simulink model "ardupilotsailboatold"  (R2022b)
settings: Solver=VariableStepAuto  StartTime=0.0  StopTime=10.0  RelTol=1e-3
values from neighbouring files (symbols this model uses):
  Ixx = 1/120 * pi * rho * L * B * T * (4*T^2 + B^2)    (= 0.835683076278)    [parameterCalculations.m]
  m = 2    [parameterCalculations.m]
  m11 = m*k11    [parameterCalculations.m]
  m22 = m*k22    [parameterCalculations.m]
  Yv = Yv * (u^2)/(U^2)    (= -23.3298597446)    [parameterCalculations.m]
undefined symbols (not defined in the file or in its folder): Waypoints
libraries: cstblocks x2, simulink x1
settings Model: Creator=ruben  LastModifiedBy=ruben

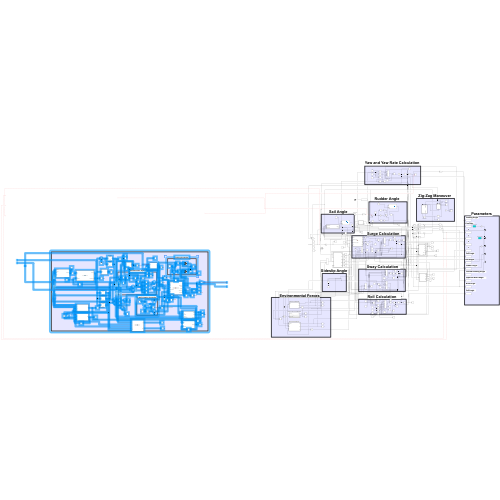
[thumbnail: Simulink's stored preview of the top-level diagram]
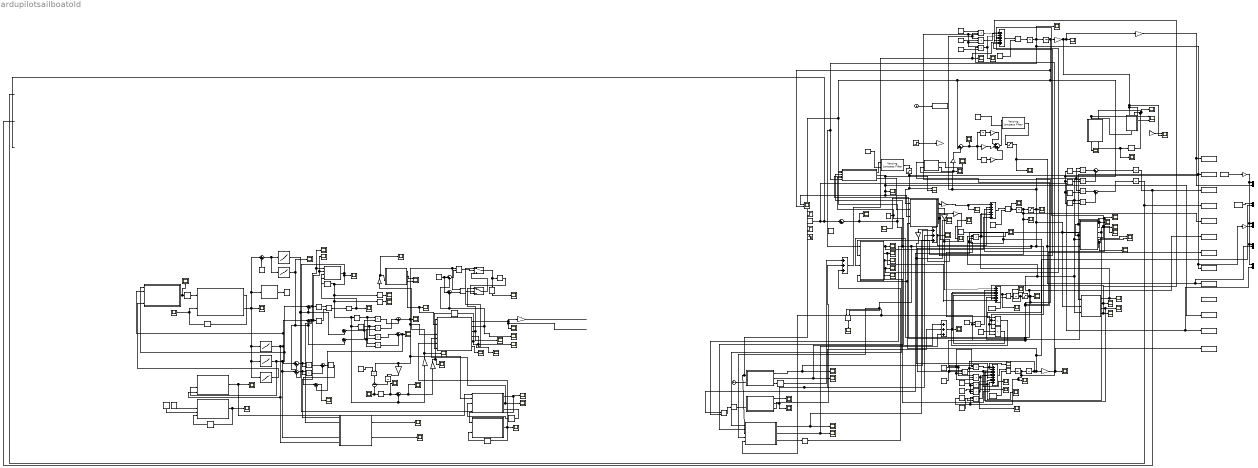
== system ardupilotsailboatold ==
  note: Yaw and Yaw Rate Calculation
  note: Surge Calculation
  note: Wave Forces and Moments
  note: Ocean Current Forces and Moments
  note: Sideslip Angle
  note: Parameters
  note: x
  note: Roll Calculation
  note: v
  note: Heading Angle
  note: u
  note: Roll Angle
  note: Sail Angle
  note: Sail Angle
  note: y
  note: Zig-Zag Maneuver
  note: Desired Heading Angle
  note: Environmental Forces
  note: Roll Angle
  note: Wind Forces and Moments
  note: Apparent Wind Angle
  note: Rudder Angle
  note: Wind Angle
  note: Sway Calculation
  note: Rudder Angle
  note: Yaw Rate
  note: Path Following Controller
  note: Tacking Controller
  note: Guidance Axis System
  Abs : Abs  SaturateOnIntegerOverflow=off
  Abs1 : Abs  SaturateOnIntegerOverflow=off
  Abs2 : Abs  SaturateOnIntegerOverflow=off
  Clock : Clock
  Clock1 : Clock
  Constant : Constant  Value=m11
  Constant1 : Constant  Value=m22
  Constant2 : Constant
  Constant27 : Constant  Value=0.1
  Constant3 : Constant  Value=-100
  Constant4 : Constant  Value=-8190/100
  Constant5 : Constant  Value=5.89/100
  Delay{1..2,4..7,9..12} (10 alike) : Delay  DelayLength=1
  Delay13 : Delay  DelayLength=1  SampleTime=2
  Delay14 : Delay  DelayLength=1  SampleTime=0.01
  Delay3 : Delay  DelayLength=1  SampleTime=2
  Derivative : Derivative
  Divide{,1..6} (7 alike) : Product  Inputs=*/
  Gain : Gain  Gain=0.9
  Gain1 : Gain  Gain=0.29
  Gain{3..4,10,17} (4 alike) : Gain  Gain=pi/180
  Gain12 : Gain  Gain=-1
  Gain{7..9,13} (4 alike) : Gain
  Gain{2,15..16,18} (4 alike) : Gain  Gain=180/pi
  Gain5 : Gain  Gain=0.01
  Gain6 : Gain  Gain=-180/pi
  Integrator{1..2,4..9} (8 alike) : Integrator
  Integrator17 : Integrator  LimitOutput=on  UpperSaturationLimit=10  LowerSaturationLimit=-10
  Integrator3 : Integrator  InitialCondition=1.3
  KS : Scope
  Kk : Scope
  Kr : Scope
  MATLAB Function : MATLAB Function  TreatAsAtomicUnit=on
  MATLAB Function1 : MATLAB Function  TreatAsAtomicUnit=on
  MATLAB Function10 : MATLAB Function  TreatAsAtomicUnit=on
  MATLAB Function11 : MATLAB Function  TreatAsAtomicUnit=on
  MATLAB Function12 : MATLAB Function  TreatAsAtomicUnit=on
  MATLAB Function13 : MATLAB Function  TreatAsAtomicUnit=on
  MATLAB Function14 : MATLAB Function  TreatAsAtomicUnit=on
  MATLAB Function15 : MATLAB Function  TreatAsAtomicUnit=on
  MATLAB Function16 : MATLAB Function  TreatAsAtomicUnit=on
  MATLAB Function18 : MATLAB Function  TreatAsAtomicUnit=on
  MATLAB Function19 : MATLAB Function  TreatAsAtomicUnit=on
  MATLAB Function2 : MATLAB Function  TreatAsAtomicUnit=on
  MATLAB Function20 : MATLAB Function  TreatAsAtomicUnit=on
  MATLAB Function21 : MATLAB Function  TreatAsAtomicUnit=on
  MATLAB Function3 : MATLAB Function  TreatAsAtomicUnit=on
  MATLAB Function4 : MATLAB Function  TreatAsAtomicUnit=on
  MATLAB Function5 : MATLAB Function  TreatAsAtomicUnit=on
  MATLAB Function6 : MATLAB Function  TreatAsAtomicUnit=on
  MATLAB Function7 : MATLAB Function  TreatAsAtomicUnit=on
  MATLAB Function8 : MATLAB Function  TreatAsAtomicUnit=on
  MATLAB Function9 : MATLAB Function  TreatAsAtomicUnit=on
  Memory : Memory
  Mux{2..6} (5 alike) : Mux  Inputs=2
  NS : Scope
  Nk : Scope
  Nr : Scope
  Product{,1..2,7..13,84..85,88} (13 alike) : Product
  Product{3..6,14..20} (11 alike) : Product  Inputs=3
  Radius of Acceptance R : Lookup_n-D  NumberOfTableDimensions=1  BreakpointsForDimension1=Waypoints.number  Table=Waypoints.R  InterpMethod=Cubic spline  ExtrapMethod=Cubic spline  InternalRulePriority=Speed  RndMeth=Simplest
  Relational Operator : RelationalOperator  Operator=<=  OutDataTypeStr=boolean  RndMeth=Simplest  InputSameDT=off
  Relational Operator1 : RelationalOperator  Operator=>  OutDataTypeStr=boolean  RndMeth=Simplest  InputSameDT=off
  Roll Axis of Rotation : Constant  Value=[ -1 0 0 ]
  Saturation : Saturate  UpperLimit=pi/6  LowerLimit=-pi/6  ZeroCross=off
  Saturation1 : Saturate  UpperLimit=1.3  LowerLimit=-1.3
  Saturation2 : Saturate  UpperLimit=pi/3  LowerLimit=-pi/3
  Saturation3 : Saturate  UpperLimit=0.1  LowerLimit=-0.1
  Scope{1,3..15,17..29,31..32,34} (30 alike) : Scope
  Scope16 : Scope  NumInputPorts=2
  Scope2 : Scope  NumInputPorts=2
  Scope30 : Scope  NumInputPorts=2
  Sine Wave : Sin  Amplitude=pi/4  Frequency=0.1  SampleTime=0
  Sqrt : Sqrt
  Step1 : Step  Time=0  After=pi-0.01  SampleTime=0
  Step2 : Step  Time=50  After=0  SampleTime=0
  Stop Simulation : Stop
  Subsystem : Subsystem
  Sum : Sum  Inputs=|+--
  Sum{1,13,15,17} (4 alike) : Sum  Inputs=|+++
  Sum{6,9..11} (4 alike) : Sum  Inputs=|+-
  Sum{7..8,14,18} (4 alike) : Sum  Inputs=|++
  Sum16 : Sum  Inputs=|--
  Sum19 : Sum  Inputs=|-+-+++++
  Sum3 : Sum  Inputs=|++++++
  Sum4 : Sum  Inputs=|+++-++++
  Sum5 : Sum  Inputs=|+-++++++++
  Tack Direction : Constant  Value=0
  Tack Left : Switch  Criteria=u2 > Threshold  SaturateOnIntegerOverflow=off  InputSameDT=off
  Tack Right : Switch  Criteria=u2 > Threshold  SaturateOnIntegerOverflow=off  InputSameDT=off
  To Workspace : ToWorkspace  VariableName=yawrate  SaveFormat=Timeseries  SampleTime=-1
  To Workspace1 : ToWorkspace  VariableName=yaw  SaveFormat=Timeseries  SampleTime=-1
  To Workspace10 : ToWorkspace  VariableName=psid  SaveFormat=Timeseries  SampleTime=-1
  To Workspace11 : ToWorkspace  VariableName=awa  SaveFormat=Timeseries  SampleTime=-1
  To Workspace12 : ToWorkspace  VariableName=wind  SaveFormat=Timeseries  SampleTime=-1
  To Workspace13 : ToWorkspace  VariableName=roll  SaveFormat=Timeseries  SampleTime=-1
  To Workspace2 : ToWorkspace  VariableName=time  SaveFormat=Timeseries  SampleTime=-1
  To Workspace3 : ToWorkspace  VariableName=x  SaveFormat=Timeseries  SampleTime=-1
  To Workspace4 : ToWorkspace  VariableName=y  SaveFormat=Timeseries  SampleTime=-1
  To Workspace5 : ToWorkspace  VariableName=u  SaveFormat=Timeseries  SampleTime=-1
  To Workspace6 : ToWorkspace  VariableName=v  SaveFormat=Timeseries  SampleTime=-1
  To Workspace7 : ToWorkspace  VariableName=phi  SaveFormat=Timeseries  SampleTime=-1
  To Workspace8 : ToWorkspace  VariableName=delta_s  SaveFormat=Timeseries  SampleTime=-1
  To Workspace9 : ToWorkspace  VariableName=delta_r  SaveFormat=Timeseries  SampleTime=-1
  Trigonometric Function{,7..8,17} (4 alike) : Trigonometry
  Trigonometric Function{1,6,9,16} (4 alike) : Trigonometry  Operator=cos
  Trigonometric Function10 : Trigonometry  Operator=atan
  Trigonometric Function15 : Trigonometry  Operator=atan
  Uniform Random Number : UniformRandomNumber  Minimum=0  Maximum=0.01  SampleTime=3  VectorParams1D=off
  Varying Lowpass Filter : cstblocks/Linear Parameter Varying/Varying Lowpass Filter  N=1
  Varying Lowpass Filter1 : cstblocks/Linear Parameter Varying/Varying Lowpass Filter  N=1
  Waypoint-1 : Sum  Inputs=|+-
  XS : Scope
  Xk : Scope
  Xr : Scope
  Yaw Axis of Rotation : Constant  Value=[ 0 1 0 ]
  Yk : Scope
  Yr : Scope
  Ys : Scope
  acceptance : Scope
  added mass : Constant  Value=m22
  added mass yaw : Constant  Value=Izz -m66
  angle : Scope
  awa : Scope  NumInputPorts=2
  awa2 : Scope
  awa3 : Scope  NumInputPorts=2
  causing windup : Gain  Gain=0
  control angle : Scope
  control angle1 : Scope
  crosstrack : Scope
  currentState : Scope
  desired heading : Step  Time=0  After=30  SampleTime=0
  distance travelled : Scope
  distanceToWaypoint : Scope
  extern : Scope
  fr2 : Constant  Value=6
  fr3 : Constant  Value=0.6
  heading : Scope
  m : Constant  Value=m
  m1 : Constant  Value=m11
  m2 : Constant  Value=m22
  m22 : Constant  Value=m22
  mass : Constant  Value=m-m11
  mass1 : Constant  Value=m-m22
  mass2 : Constant  Value=Ixx
  nextTackType : Scope
  p2 : Constant  Value=Yv
  p_w : Scope
  "pathFollowingController+waypoint " : Scope
  pathfollowingcontroller : Scope
  pathtrajectory : Scope
  pathx : Scope
  pathy : Scope
  rudder and psi : Scope  NumInputPorts=2
  rudder angle{,1..2,4} (4 alike) : Scope
  rudder angle3 : Scope  NumInputPorts=3
  state : Scope
  tack required : Scope
  tackDistance : Scope
  tackHeading : Scope
  tackLeft : Scope
  tackRight : Scope
  tackSide : Scope
  tackside : Scope
  tan : Scope
  theta : Scope
  track : Scope
  trackx distance to waypoint : Scope
  uc : Scope
  vc : Scope
  wayPointHeading : Scope
  waypoint : Scope
  wi_u : Scope
  wi_v : Scope
  wind Velocity : Constant  Value=10
  wind direction : Constant  Value=pi/2-0.01
  wu : Scope
  wv : Scope
  wv1 : Scope
  x-coordinates : Lookup_n-D  NumberOfTableDimensions=1  BreakpointsForDimension1=Waypoints.number  Table=Waypoints.x  InterpMethod=Cubic spline  ExtrapMethod=Cubic spline  InternalRulePriority=Speed  RndMeth=Simplest
  x-coordinates1 : Lookup_n-D  NumberOfTableDimensions=1  BreakpointsForDimension1=Waypoints.number  Table=Waypoints.x  InterpMethod=Cubic spline  ExtrapMethod=Cubic spline  InternalRulePriority=Speed  RndMeth=Simplest
  x1 : Scope
  x2 : Scope
  xd = xp+xr : Sum  Inputs=|++
  xh : Sum  Inputs=|+-
  xr : Trigonometry  Operator=atan
  xsd : Sum  Inputs=|+-
  xtrack : Sum  Inputs=|++
  xtrack distance to waypoint : Sum  Inputs=|+-
  y-coordinates : Lookup_n-D  NumberOfTableDimensions=1  BreakpointsForDimension1=Waypoints.number  Table=Waypoints.y  InterpMethod=Cubic spline  ExtrapMethod=Cubic spline  InternalRulePriority=Speed  RndMeth=Simplest
  y-coordinates1 : Lookup_n-D  NumberOfTableDimensions=1  BreakpointsForDimension1=Waypoints.number  Table=Waypoints.y  InterpMethod=Cubic spline  ExtrapMethod=Cubic spline  InternalRulePriority=Speed  RndMeth=Simplest
  y11 : Scope
  yh : Sum  Inputs=|+-
  ysd : Sum  Inputs=|+-
  ytrack : Sum  Inputs=|-+
  z - y1 : Gain  Gain=-1
  z - y2 : Gain  Gain=-1
  wires:
  ? -> Sum/1
  ? -> Scope30/2
  MATLAB Function2/2(nextState) -> rudder angle1/1, Delay14/1
  Integrator6/1 -> Product2/2, Product17/3, Product17/2, MATLAB Function/4(phi), MATLAB Function21/4(phi), Mux6/2, Gain6/1
  MATLAB Function1/2(alpha_aw) -> Scope2/2, awa/1, MATLAB Function/3(apparent_wind_angle), Scope7/1, To Workspace11/1
  MATLAB Function21/1(Xh) -> Sum3/6, Scope18/1
  Constant3/1 -> Product6/2
  MATLAB Function21/5(Frh) -> Scope12/1
  Integrator9/1 -> Product20/2, Abs/1, Product6/1, Scope26/1, Integrator6/1
  Product6/1 -> Sum5/6
  Product14/1 -> Sum3/4, Scope8/1
  Sum5/1 -> Divide4/1
  MATLAB Function21/4(Nh) -> Sum19/8, Scope21/1
  Divide3/1 -> Scope3/1
  Product16/1 -> Sum4/5
  MATLAB Function14/2(wv) -> Sum15/1, wv/1
  MATLAB Function1/3(V_aw) -> MATLAB Function/2(apparent_velocity)
  Saturation1/1 -> MATLAB Function16/2(u), MATLAB Function13/2(u), Divide2/2, MATLAB Function1/3(u), MATLAB Function15/4(u), Divide3/2, Product5/2, Product3/3, Product4/2, Product16/1, Product15/2, Product18/2, Product19/1, MATLAB Function19/2(U), Product/1, Product8/1, Scope4/1
  Delay14/1 -> rudder angle4/1, MATLAB Function20/2(state), MATLAB Function2/2(currentState)
  Divide4/1 -> Integrator9/1
  Product4/1 -> Scope15/1, Sum5/2
  Abs/1 -> Product6/3
  Saturation3/1 -> Product14/2, Product1/1, Product9/1, MATLAB Function13/3(v), MATLAB Function16/3(v), To Workspace6/1, MATLAB Function21/3(v), To Workspace7/1, MATLAB Function19/1(v), MATLAB Function15/5(v), Divide3/1, Product7/2, Product3/2, Product5/3, Product4/3, MATLAB Function1/4(v), Product20/1, Product19/3, Product18/3, Scope5/1
  wind direction/1 -> Mux5/2, To Workspace12/1, Sum18/1
  z - y2/1 -> Mux2/2
  MATLAB Function13/4(Nr) -> Sum19/4, Nr/1
  Product18/1 -> Sum19/1
  Trigonometric Function7/1 -> Product8/2
  Trigonometric Function10/1 -> Subsystem/2(angle of attack)
  Divide1/1 -> Integrator4/1
  Integrator4/1 -> Scope25/1, Saturation3/1
  Yaw Axis of Rotation/1 -> z - y1/1
  Gain7/1 -> KS/1, Sum5/7
  Roll Axis of Rotation/1 -> Mux6/1
  Sum18/1 -> MATLAB Function1/2(wind_direction), MATLAB Function15/1(windDirect), Scope24/1
  Gain9/1 -> XS/1, Sum3/1
  MATLAB Function20/1(y) -> rudder angle3/1, MATLAB Function2/1(r)
  Gain18/1 -> rudder and psi/1
  Saturation/1 -> MATLAB Function13/4("delta_r "), Mux3/2, To Workspace9/1, rudder angle/1
  MATLAB Function14/3(wr) -> Delay9/1
  Gain17/1 -> Mux4/2, To Workspace1/1
  MATLAB Function21/3(Kh) -> Scope20/1, Sum5/10
  Sum6/1 -> Integrator1/1
  Gain16/1 -> rudder and psi/2, MATLAB Function20/1(psi), rudder angle3/3, Gain17/1, Scope30/1
  Integrator1/1 -> To Workspace4/1
  MATLAB Function16/2(Yk) -> Sum4/7, Yk/1
  Sum13/1 -> Sum19/7, extern/1
  MATLAB Function16/1(Xk) -> Sum3/5, Xk/1
  MATLAB Function16/3(Kk) -> Sum5/3, Kk/1
  Product17/1 -> Sum5/9, Scope27/1
  MATLAB Function19/2(y1) -> Gain12/1, Scope29/1
  MATLAB Function13/2(Yr) -> Yr/1, Sum4/6
  MATLAB Function16/4(Nk) -> Sum19/6, Nk/1
  Integrator3/1 -> MATLAB Function21/2(u), Scope9/1, To Workspace5/1, Saturation1/1
  MATLAB Function21/2(Yh) -> Sum4/8, Scope19/1
  MATLAB Function/5(awa) -> Scope23/1
  Varying Lowpass Filter/1 -> Saturation/1
  MATLAB Function13/1(Xr) -> Xr/1, Sum3/3
  Gain13/1 -> NS/1
  added mass yaw/1 -> Divide5/2
  Integrator8/1 -> awa/2, Trigonometric Function1/1, Trigonometric Function6/1, Trigonometric Function7/1, Trigonometric Function/1, MATLAB Function1/1(psi), MATLAB Function15/3(psi), MATLAB Function14/1(beta), Sum/2, Gain16/1
  z - y1/1 -> Mux5/1, Mux3/1, Mux2/1, Mux4/1
  Constant/1 -> Product5/1, Product3/1
  MATLAB Function14/1(wu) -> Sum17/1, wu/1  "1"
  Sum/1 -> Scope10/1, Derivative/1, Integrator5/1, Gain/1
  Product3/1 -> Sum5/1, Scope13/1
  m2/1 -> Product20/3
  Product5/1 -> Scope14/1, Sum5/5
  Sum19/1 -> Divide5/1
  Sum15/1 -> Sum4/3, wv1/1
  Product20/1 -> Scope34/1, Sum19/3
  Gain5/1 -> Sum1/1
  Product2/1 -> Scope6/1, Sum5/8
  Constant5/1 -> Product17/1
  Product19/1 -> Sum19/2
  MATLAB Function2/1(y) -> rudder angle2/1
  Sum17/1 -> Sum3/2, Scope11/1
  Divide/1 -> Scope1/1, Integrator3/1
  MATLAB Function15/2(wi_v) -> Sum15/3, wi_v/1
  fr2/1 -> Varying Lowpass Filter/2
  Subsystem/1(uc) -> uc/1
  Sum1/1 -> Varying Lowpass Filter/1
  Divide5/1 -> Integrator7/1
  MATLAB Function13/5(delta_r) -> Scope32/1, Scope16/1
  Gain6/1 -> Scope22/1, To Workspace13/1
  mass1/1 -> Divide1/2
  MATLAB Function19/1(y) -> Scope28/1
  MATLAB Function/1(Xs) -> Gain9/1
  Gain1/1 -> Sum1/3
  Gain8/1 -> Sum4/1, Ys/1
  Varying Lowpass Filter1/1 -> Saturation2/1
  added mass/1 -> Product16/2
  desired heading/1 -> Gain4/1
  MATLAB Function15/3(wi_r) -> Delay10/1
  Subsystem/3(rc) -> Sum13/2
  MATLAB Function1/1(y) -> Varying Lowpass Filter1/1
  Clock1/1 -> MATLAB Function14/2(t)
  m1/1 -> Product19/2
  Gain/1 -> Sum1/2
  Integrator2/1 -> To Workspace3/1
  MATLAB Function15/1(wi_u) -> wi_u/1, Sum17/3
  mass/1 -> Divide/2
  Delay9/1 -> Sum13/1
  p2/1 -> Product7/1
  Product7/1 -> Sum4/2
  Sum7/1 -> Integrator2/1
  Product8/1 -> Sum7/1
  m/1 -> Product14/1, Product15/1
  Derivative/1 -> Gain1/1
  Integrator5/1 -> Gain5/1
  Sum3/1 -> Divide/1
  Subsystem/2(vc) -> vc/1, Sum15/2, Sum17/2
  Constant4/1 -> Product2/1
  Product1/1 -> Sum6/2
  Clock/1 -> To Workspace2/1
  MATLAB Function/4(Ns) -> Gain13/1, Sum19/5
  Divide2/1 -> Trigonometric Function10/1
  Constant1/1 -> Product4/1
  Product9/1 -> Sum7/2
  Sum4/1 -> Scope17/1, Divide1/1
  Integrator7/1 -> MATLAB Function21/1(r), MATLAB Function1/6(r), MATLAB Function16/1(r), Product16/3, Product15/3, Divide2/1, Product14/3, MATLAB Function13/1(r), To Workspace/1, Scope31/1, Integrator8/1
  fr3/1 -> Varying Lowpass Filter1/2
  m22/1 -> Product18/1
  Product/1 -> Sum6/1
  Product15/1 -> Sum4/4
  MATLAB Function13/6(alpha_a) -> Scope16/2
  mass2/1 -> Divide4/2
  Trigonometric Function1/1 -> Product/2
  Saturation2/1 -> MATLAB Function/1(delta_s), Scope2/1, To Workspace8/1, z - y2/1
  Gain12/1 -> Sum/3
  Trigonometric Function/1 -> Product1/2
  MATLAB Function/3(Ks) -> Gain7/1
  MATLAB Function13/3(Kr) -> Kr/1, Sum5/4
  MATLAB Function/2(Ys) -> Gain8/1
  Delay10/1 -> Sum13/3
  wind Velocity/1 -> MATLAB Function15/2(V_w), MATLAB Function1/5(wind_velocity)
  Trigonometric Function6/1 -> Product9/2
  ? -> yh/1, MATLAB Function6/2(yw), MATLAB Function5/4(yBoat), MATLAB Function11/4(ys), MATLAB Function12/2(ys), Delay5/1
  Delay3/1 -> MATLAB Function18/2(currentState)
  Gain10/1 -> MATLAB Function7/2(psi), awa2/1
  Delay13/1 -> MATLAB Function9/3(currentState)
  MATLAB Function3/5(nextTackType) -> nextTackType/1, Delay12/1
  MATLAB Function18/1(nextState) -> tackside/1, Delay3/1, MATLAB Function3/6(zone)
  Integrator17/1 -> Sum16/2
  Abs1/1 -> Divide6/1
  MATLAB Function3/2(tackDistance) -> tackDistance/1, Sum10/2, Sum14/2
  Delay7/1 -> MATLAB Function8/4(us)
  Product85/1 -> ytrack/1
  Delay11/1 -> tackHeading/1
  Trigonometric Function16/1 -> Product11/1, Product84/1
  MATLAB Function7/2(w) -> awa3/1
  Sum14/1 -> Relational Operator1/2
  MATLAB Function4/2(currentWaypoint) -> MATLAB Function10/1(state), Waypoint-1/1, waypoint/1, Radius of Acceptance R/1, x-coordinates/1, y-coordinates/1
  Gain2/1 -> pathtrajectory/1, MATLAB Function3/1(pathTrajectory)
  Radius of Acceptance R/1 -> MATLAB Function5/5(R)
  yh/1 -> Product85/2, Product11/2
  Delay12/1 -> MATLAB Function3/7(currentTackType)
  MATLAB Function3/6(currentState) -> currentState/1
  y-coordinates/1 -> MATLAB Function11/6(ycw), MATLAB Function6/4(ywp), MATLAB Function5/2(yWaypoint), ysd/1, Sum9/1
  Waypoint-1/1 -> x-coordinates1/1, y-coordinates1/1
  MATLAB Function3/1(y) -> heading/1, Gain3/1
  MATLAB Function11/2(theta) -> theta/1
  MATLAB Function7/3(p) -> awa3/2
  xr/1 -> xd = xp+xr/1, pathfollowingcontroller/1
  Product12/1 -> Sum8/1
  Product10/1 -> xtrack/1
  Trigonometric Function9/1 -> pathx/1
  ? -> MATLAB Function3/3(WA), MATLAB Function7/1(wa)
  ? -> MATLAB Function9/4(windDirection)
  y-coordinates1/1 -> yh/2, ysd/2, Sum9/2, x2/1
  x-coordinates1/1 -> Sum11/2, xh/2, xsd/2
  Trigonometric Function17/1 -> Product10/1, Product85/1
  Sum16/1 -> xr/1, tan/1
  Trigonometric Function15/1 -> control angle1/1, MATLAB Function8/3(u)
  ysd/1 -> y11/1, MATLAB Function8/2(y1), Abs2/1, MATLAB Function11/2(yw)
  MATLAB Function3/4(tackRight) -> Tack Right/1, tackRight/1
  Constant2/1 -> Waypoint-1/2
  MATLAB Function9/1(angle) -> angle/1, MATLAB Function18/1(angle)
  Delay5/1 -> MATLAB Function12/4(y)
  xd = xp+xr/1 -> "pathFollowingController+waypoint "/1, Gain2/1
  MATLAB Function9/3(nextState) -> Delay13/1
  Delay1/1 -> MATLAB Function4/1(R)
  xsd/1 -> MATLAB Function11/1(xw), MATLAB Function8/1(x1), x1/1, Abs1/1
  xh/1 -> Product84/2, Product10/2
  Delay2/1 -> MATLAB Function4/2(currentState), state/1
  ytrack/1 -> MATLAB Function3/4(xtrack), Product88/2, causing windup/1, MATLAB Function9/2(xtrack), crosstrack/1, Relational Operator1/1, Relational Operator/1
  ? -> xh/1, MATLAB Function11/3(xs), MATLAB Function12/1(xs), Delay4/1, MATLAB Function6/1(xw), MATLAB Function5/3(xBoat)
  Sum10/1 -> Relational Operator/2
  Relational Operator/1 -> Tack Right/2
  Delay6/1 -> MATLAB Function12/5("dist ")
  MATLAB Function5/1(acceptance) -> acceptance/1, Delay1/1
  Sum8/1 -> Sqrt/1
  Tack Left/1 -> Tack Right/3
  MATLAB Function6/1(y) -> MATLAB Function9/1(dist), distanceToWaypoint/1
  MATLAB Function9/2(tack) -> MATLAB Function3/5(indirectTackSide), tackSide/1
  MATLAB Function10/1(y) -> Stop Simulation/1
  Delay4/1 -> MATLAB Function12/3(x)
  Sum9/1 -> Product12/1, Product12/2
  Product13/1 -> Sum8/2
  Trigonometric Function8/1 -> pathy/1
  Sum11/1 -> Product13/2, Product13/1
  x-coordinates/1 -> MATLAB Function6/3(xwp), MATLAB Function11/5(xcw), Sum11/1, xsd/1, MATLAB Function5/1(xWaypoint)
  Constant27/1 -> Product88/1
  Memory/1 -> Tack Left/3
  Relational Operator1/1 -> Tack Left/2
  Tack Right/1 -> Memory/1, Delay11/1
  MATLAB Function3/3(tackLeft) -> tackLeft/1, Tack Left/1
  Product88/1 -> Sum16/1
  Sqrt/1 -> xtrack distance to waypoint/1
  MATLAB Function11/1(p_w) -> p_w/1
  MATLAB Function4/1(nextState) -> Delay2/1
  xtrack distance to waypoint/1 -> trackx distance to waypoint/1
  MATLAB Function12/1(dist) -> distance travelled/1, Delay6/1
  Abs2/1 -> Divide6/2
  xtrack/1 -> xtrack distance to waypoint/2, track/1
  Gain15/1 -> Gain10/1, wayPointHeading/1
  MATLAB Function8/1(y) -> Trigonometric Function8/1, Trigonometric Function9/1, Trigonometric Function17/1, xd = xp+xr/2, Gain15/1, Trigonometric Function16/1, Delay7/1, control angle/1, MATLAB Function9/5(wayPointHeading)
  Product84/1 -> ytrack/2
  MATLAB Function7/1(y) -> MATLAB Function3/2(tack), tack required/1
  Divide6/1 -> Trigonometric Function15/1
  Tack Direction/1 -> Sum14/1, Sum10/1
  Gain3/1 -> ?
  Product11/1 -> xtrack/2
  causing windup/1 -> Integrator17/1

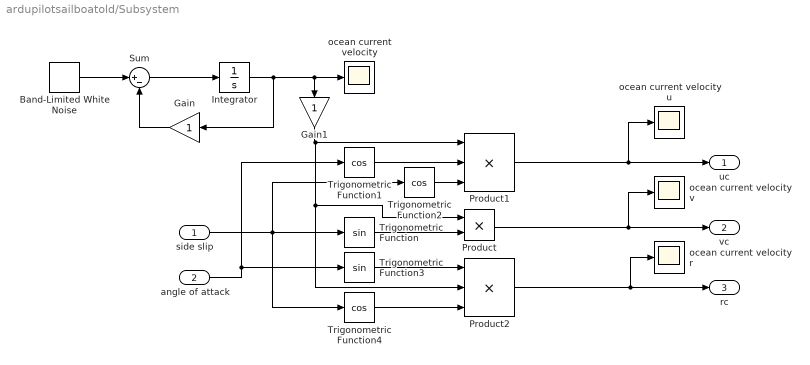
== system ardupilotsailboatold/Subsystem ==
  side slip : Inport
  angle of attack : Inport  Port=2
  Band-Limited White Noise : simulink/Sources/Band-Limited White Noise  Cov=[0.03]  Ts=1  seed=[23341]
  Gain : Gain
  Gain1 : Gain
  Integrator : Integrator
  Product : Product
  Product1 : Product  Inputs=3
  Product2 : Product  Inputs=3
  Sum : Sum  Inputs=|+-
  Trigonometric Function : Trigonometry
  Trigonometric Function1 : Trigonometry  Operator=cos
  Trigonometric Function2 : Trigonometry  Operator=cos
  Trigonometric Function3 : Trigonometry
  Trigonometric Function4 : Trigonometry  Operator=cos
  ocean current velocity : Scope
  ocean current velocity r : Scope
  ocean current velocity u : Scope
  ocean current velocity v : Scope
  uc : Outport
  vc : Outport  Port=2
  rc : Outport  Port=3
  wires:
  Sum/1 -> Integrator/1
  Band-Limited White Noise/1 -> Sum/1
  Integrator/1 -> ocean current velocity/1, Gain1/1, Gain/1
  Gain/1 -> Sum/2
  Trigonometric Function/1 -> Product/2
  side slip/1 -> Trigonometric Function4/1, Trigonometric Function2/1, Trigonometric Function/1
  Product/1 -> ocean current velocity v/1, vc/1
  Trigonometric Function2/1 -> Product1/3
  Trigonometric Function1/1 -> Product1/2
  Product1/1 -> ocean current velocity u/1, uc/1
  Trigonometric Function3/1 -> Product2/1
  Trigonometric Function4/1 -> Product2/3
  angle of attack/1 -> Trigonometric Function3/1, Trigonometric Function1/1
  Product2/1 -> rc/1, ocean current velocity r/1
  Gain1/1 -> Product1/1, Product2/2, Product/1

== matlab function ardupilotsailboatold/MATLAB Function15 ==
  data: windDirect input; wi_u output; wi_v output; wi_r output; V_w input; psi input; u input; v input
function [wi_u,wi_v,wi_r] = WindForcesandMoments(windDirect,V_w,psi,u,v)
% Air density (kg/m^2)
rho = 1.225;

% Ship Size
L = 2;
B = 0.125;
T = 0.4;

% centroids above the water line of the frontal and lateral projected areas
H_fw = T - 1.2;
H_lw = T - 1.2;
A_fw = B * H_fw;
A_lw = L * H_lw;


% Symmetrical Ship Coeff
c_x = 0.7;
c_y = 0.825;
c_r = 0.125;

% Wind Velocities in x- and y-coordinates
u_w = V_w * cos(windDirect - psi);
v_w = V_w * sin(windDirect - psi);

% Relative wind velocities
u_rw = u - u_w;
v_rw = v - v_w;

% Relative Wind Velocity and direction
V_rw = sqrt(u_rw^2 + v_rw^2);
gamma_rw = -atan(v_rw/u_rw);

% Wind Coeff
C_x = -c_x * cos(gamma_rw);
C_y = c_y * sin(gamma_rw);
C_r = c_r * sin(2*gamma_rw);

% Wind Forces and Moments
wi_u = 0.5 * rho * V_rw *  C_x * A_fw * 10^(-2);
wi_v = 0.5 * rho * V_rw *  C_y * A_lw * 10^(-2);
wi_r = 0.5 * rho * V_rw *  C_r * A_lw * 10^(-2);

== matlab function ardupilotsailboatold/MATLAB Function16 ==
  data: r input; u input; Xk output; v input; Yk output; Kk output; Nk output
function [Xk,Yk,Kk,Nk] = keelForce(r,u,v)
%Parameters
keel_width = 8;
keel_length = 45;
rho_w = 1025;
area = keel_width * keel_length * 10^(-4);
velocity = sqrt(v^2+u^2);
l3 = 0.1;
h2 = 0.275;
yk=0;
xk=0.1;
zk=0.25;

% Calculate Angle of Attack
v_aku = -u + r*yk;
v_akv = -v - r*xk + 0*zk;
alpha_ak = atan2(real(v_akv),real(-v_aku));
alpha = alpha_ak;

% Lift and Drag Coeff
[lc, dc] = keelcoef(alpha);

% Calculate Lift and Drag Force
lift_force = 0.5 * rho_w * area * lc * (v_aku^2+v_akv^2);
drag_force = 0.5 * rho_w * area * dc * (v_aku^2+v_akv^2);

Xk = (-lift_force * sin(alpha_ak) + drag_force * cos(alpha_ak));
Yk = (-lift_force * cos(alpha_ak) - drag_force * sin(alpha_ak));
Kk = -(-lift_force*cos(alpha_ak)-drag_force*sin(alpha_ak))*zk;
Nk = -(lift_force*cos(alpha_ak)+drag_force*sin(alpha_ak))*xk;



%------------------------------------------------------------------------------------------------------------------------------
function [Clk,Cdk] = keelcoef(attack)
% generate a lookup table for the lift/drag coefficients for the sail
% and compute Cls/Cds from the lookup table using interpolation.

% lookup table
xdata = linspace(-pi,pi,73); % every 5 degrees
xdata = xdata/pi*180;

% lift curve
yl = fliplr([0 0.425 0.74 ...
    0.94 1.1 1.17 1.19 1.16 1.12 1.07 0.99 0.92 0.84 0.74 0.63 0.49 0.345 0.185])*(-1);
yldata = [fliplr([0 0.425 0.74 ...
    0.94 1.1 1.17 1.19 1.16 1.12 1.07 0.99 0.92 0.84 0.74 0.63 0.49 0.345 0.185 0 yl])*(-1) ...
    [0.425 0.74 ...
    0.94 1.1 1.17 1.19 1.16 1.12 1.07 0.99 0.92 0.84 0.74 0.63 0.49 0.345 0.185 0 yl]];

% drag curve
yd = fliplr([0 0.04 0.07 ...
    0.1 0.17 0.3 0.49 0.76 0.98 1.19 1.34 1.5 1.65 1.77 1.88 1.96 2.01 2.05]);
yddata = [fliplr([0 0.04 0.07 ...
    0.1 0.17 0.3 0.49 0.76 0.98 1.19 1.34 1.5 1.65 1.77 1.88 1.96 2.01 2.05 2.09 yd])...
    [0.04 0.07 ...
    0.1 0.17 0.3 0.49 0.76 0.98 1.19 1.34 1.5 1.65 1.77 1.88 1.96 2.01 2.05 2.09 yd]];

% fit the input angle of attack into the interval [-pi,pi]
if attack > pi
    attack = mod(attack+pi,2*pi) - pi;
else
    if attack < -pi
        attack = mod(attack-pi,-2*pi) + pi;
    end
end

% interpolation
attack = attack/pi*180;
Clk = interp1(xdata,yldata,attack,'pchip');
Cdk = interp1(xdata,yddata,attack,'pchip');


%------------------------------------------------------------------------------------------------------------------------------
function F = resistancehull(alpha_a)

xdata = linspace(0,6,13); % every 0.5m/s
ydata = [0 0.15 0.35 0.5 0.675 0.825 1.175 1.4 2 4.85 9.85 18.46 27.5]*1000;

% interpolation
if alpha_a <= 6
    F = interp1(xdata,ydata,alpha_a,'pchip');
else
    F = interp1(xdata,ydata,alpha_a,'pchip','extrap');
end

== matlab function ardupilotsailboatold/MATLAB Function10 ==
  data: state input; y output
function y = stopSimulation(state)
if state== 6
    y=1;
else
    y=0;
end

== matlab function ardupilotsailboatold/MATLAB Function19 ==
  data: y output; v input; U input; y1 output
function [y,y1]     = beta(v,U)
% Beta Reference Angle
y=0;
y1 = real(asin(complex(v/U)));

== matlab function ardupilotsailboatold/MATLAB Function20 ==
  data: y output; psi input; state input
function y      = zigzagPsi(psi,state)
% Beta Reference Angle
if psi<-15 && state == 0
    y=1;
elseif psi>15 && state == 1
    y=1;
else 
    y=0;
end

== matlab function ardupilotsailboatold/MATLAB Function21 ==
  data: r input; u input; Xh output; v input; Yh output; Kh output; Nh output; Frh output; phi input
function [Xh,Yh,Kh,Nh,Frh] = hullForce(r,u,v,phi)
yh=0;
zh=-0.1;
xh=0;
% from the hull
v_ahu = -u + r*yh;
v_ahv = (-v-r*xh + 0*zh)/cos(0);
v_ah = sqrt(v_ahu^2+v_ahv^2);
alpha_ah = atan2(real(v_ahv),real(-v_ahu));
Frh = resistancehull(v_ah);

Xh = Frh*cos(alpha_ah)*2;
Yh = -Frh*sin(alpha_ah)*cos(phi)*100;
Kh = Frh*sin(alpha_ah)*cos(phi)*zh;
Nh = -Frh*sin(alpha_ah)*cos(0)*xh;
%D_hull = [Frh*cos(alpha_ah);-Frh*sin(alpha_ah)*cos(phi); Frh*sin(alpha_ah)*cos(phi)*par.zh; -Frh*sin(alpha_ah)*cos(phi)*par.xh];


function F = resistancehull(alpha_a)

xdata = linspace(0,0.15,13); % every 0.1m/s
ydata = [0 0.075 0.175 0.25 0.3375 0.4125 0.5875 0.7 1 2.425 4.925 9.23 13.75]*0.08;

% interpolation
if alpha_a <= 0.15
    F = interp1(xdata,ydata,alpha_a,'pchip');
else
    F = interp1(xdata,ydata,alpha_a,'pchip','extrap');
end

== matlab function ardupilotsailboatold/MATLAB Function11 ==
  data: xw input; yw input; xs input; p_w output; ys input; xcw input; ycw input; theta output
function [p_w,theta] = passedWaypoint(xw,yw,xs,ys,xcw,ycw)
% Checking is sailboat has passed waypoint while sailing into the wind
if (ys-ycw)~= 0
theta = atan(abs(xs-xcw)/abs(ys-ycw));
else 
    theta=0;
end

p_w=0;
if xw>0 
% Angle between sail
    if (xcw-xs)<0 
        % Waypoint passed in x positive
        p_w=1;
        if(ycw-ys)<0
            % Waypoint passed in both x and y positive direction
            theta = pi + theta;
        else
            % Waypoint passed in positive x and negative y
            theta = -theta;
        end
    end 
else
    if(xcw-xs)>0 
        % Waypoint passed in x negative
        p_w=1;
        if(ycw-ys)>0
           % Waypoint passed in both x and y negative direction
        else
           % Waypoint passed in negative x and positive y
           theta= pi - theta;
        end
   end
end

== matlab function ardupilotsailboatold/MATLAB Function12 ==
  data: xs input; ys input; x input; y input; dist input; dist output
function dist   = travelDistance(xs,ys,x,y,dist)
% Distance Sailboat travelled

dist = dist + sqrt((xs-x)^2+(ys-y)^2);

== matlab function ardupilotsailboatold/MATLAB Function18 ==
  data: angle input; nextState output; currentState input
function nextState    = tack_Side(angle,currentState)
% Calculate when to tack back to waypoint

switch currentState
    case 1
        % In zone 1 can go to zone 2 and 4
        if angle < 0
            nextState=4;
        elseif angle > 15
            nextState=2;
        else 
            nextState=1;
        end
    case 2
       % In zone 2 can go to zone 3 and 1
        if angle < 15
            nextState=1;
        elseif angle > 30
            nextState=3;
        else 
            nextState=2;
        end
    case 3
        % In zone 3 can go to zone 2
        if angle < 30
            nextState=2;
        else 
            nextState=3;
        end
    case 4
       % In zone 4 can go to zone 5 and 1
        if angle > 0
            nextState=1;
        elseif angle < -15
            nextState=5;
        else 
            nextState=4;
        end
    case 5
       % In zone 5 can go to zone 6 and 4
        if angle < -30
            nextState=6;
        elseif angle >-15
            nextState=4;
        else
            nextState=5;
        end
    case 6
        % In zone 6 can go to zone 5
        if angle > -30
            nextState=5;
        else 
            nextState=6;
        end
    otherwise
        nextState=1;

end

== matlab function ardupilotsailboatold/MATLAB Function3 ==
  data: pathTrajectory input; y output; tack input; tackDistance output; tackLeft output; tackRight output; WA input; xtrack input; nextTackType output; indirectTackSide input; zone input; currentTackType input; currentState output
function [y,tackDistance, tackLeft,tackRight,nextTackType,currentState]  = headingController(pathTrajectory,tack,WA,xtrack,indirectTackSide,zone,currentTackType)
% Heading State Machine

% Type of Tacks
% Direct = 1
% Indirect = 2
% Zones = 3

tackDistance = 10;
if tack==0
    currentState = 0;
else
    % Switch between Direct and Indirect Tack and Zone Tack
    currentState = 1;
    
end
switch currentState
    
    % Normail State 
    case 0
        y = pathTrajectory;
        nextTackType=1;
        tackLeft=0;
        tackRight=0;

    % Direct Tacking State
    case 1
       switch currentTackType
           case 1
               y=-WA*180/pi+45;
               tackRight=1;
               tackLeft=0;
               if(xtrack>tackDistance)
                   nextTackType=0;
               else
                   nextTackType=1;
               end
               
           case 0 
               y=-WA*180/pi-45;
               tackRight=0;
               tackLeft=1;
               if (xtrack<-tackDistance)
                   nextTackType=1;
               else 
                   nextTackType=0;
               end
           otherwise
               nextTackType=1;
               y=WA*180/pi+45;
               tackLeft=1;
               tackRight=0;
       end
    
    % Indirect Tacking State
    case 2
        if indirectTackSide==0
             y=WA*180/pi+45;
        else
             y=WA*180/pi-45;
        end
        nextTackType=1;
        tackLeft=0;
        tackRight=0;

    % Zone Tacking State
    case 3
        switch zone
            case 1
                if currentTackType==0
                    tackLeft=1;
                    tackRight=0;
                    y=WA*180/pi-45;
                    nextTackType=0;
                else
                    tackLeft=0;
                    tackRight=1;
                    y=WA*180/pi+45;
                    nextTackType=1;
                end

            case 2
                if currentTackType==0
                    tackLeft=1;
                    tackRight=0;
                    y=WA*180/pi-45;
                    nextTackType=0;
                else
                    tackLeft=0;
                    tackRight=1;
                    y=WA*180/pi+45;
                    nextTackType=1;
                end

            case 3
                % If boat is forced in zone 3 sail past lay lines and only
                % when one has passed the lay lines sail to waypoint
                y = pathTrajectory;
                tackLeft=1;
                nextTackType=0;
                tackRight=0;
            
            case 4
                if currentTackType==0
                    tackLeft=1;
                    tackRight=0;
                    y=WA*180/pi-45;
                    nextTackType=0;
                else
                    tackLeft=0;
                    tackRight=1;
                    y=WA*180/pi+45;
                    nextTackType=1;
                end

            case 5
                if currentTackType==0
                    tackLeft=1;
                    tackRight=0;
                    y=WA*180/pi-45;
                    nextTackType=0;
                else
                    tackLeft=0;
                    tackRight=1;
                    y=WA*180/pi+45;
                    nextTackType=1;
                end

            case 6
                % Same as zone 3 just opposite tack
                y = pathTrajectory;
                tackLeft=0;
                nextTackType=1;
                tackRight=1;

            otherwise
                y = pathTrajectory;
                nextTackType=0;
                tackLeft=1;
                tackRight=0;
        end

    otherwise
        y=0;
        nextTackType=2;
        tackLeft=0;
        tackRight=0;

end
if currentState==3
    if tackLeft==1
         y=WA*180/pi-45;
         nextTackType=0;
    else
         y=WA*180/pi+45;
         nextTackType=1;
    end
end

== matlab function ardupilotsailboatold/MATLAB Function4 ==
  data: R input; nextState output; currentWaypoint output; currentState input
function [nextState,currentWaypoint]  = wayPointController(R,currentState)
% Waypoint switching
% With each added waypoint another case should be added
switch currentState
    % First waypoint
    case 0
        % Check if waypoint lies within radius of acceptance
        if(R==1)
            % Switch current Waypoint to next waypoint
            nextState=1;
            currentWaypoint=1;
        % Waypoint not reached
        else
            nextState=0;
            currentWaypoint=0;
        end
    case 1
        % Check if waypoint lies within radius of acceptance
        if(R==1)
            % Switch current Waypoint to next waypoint
            nextState=2;
            currentWaypoint=2;
       % Waypoint not reached
       else
            nextState=currentState;
            currentWaypoint=1;
       end
    case 2
       % Check if waypoint lies within radius of acceptance
       if(R==1)
            % Switch current Waypoint to next waypoint
            nextState=3;
            currentWaypoint=3;
       % Waypoint not reached
       else
            nextState=currentState;
            currentWaypoint=2;
       end
     case 3
       % Check if waypoint lies within radius of acceptance
       if(R==1)
            % Switch current Waypoint to next waypoint
            nextState=4;
            currentWaypoint=4;
       % Waypoint not reached 
       else
            nextState=currentState;
            currentWaypoint=3;
       end
     case 4
       % Check if waypoint lies within radius of acceptance
       if(R==1)
            % Switch current Waypoint to next waypoint
            nextState=5;
            currentWaypoint=5;
       % Waypoint not reached
       else
            nextState=currentState;
            currentWaypoint=4;
       end
       case 5
       % Check if waypoint lies within radius of acceptance
       if(R==1)
            % Switch current Waypoint to next waypoint
            nextState=0;
            currentWaypoint=0;
       % Waypoint not reached
       else
            nextState=currentState;
            currentWaypoint=5;
       end
    otherwise
        nextState=0;
        currentWaypoint=0;
end

== matlab function ardupilotsailboatold/MATLAB Function5 ==
  data: xWaypoint input; yWaypoint input; xBoat input; yBoat input; R input; acceptance output
function acceptance   = circleOfAcceptanceController(xWaypoint,yWaypoint,xBoat,yBoat,R)
    if (sqrt((abs(xWaypoint-xBoat))^2+(abs(yWaypoint-yBoat))^2)<R)
        acceptance=1;
    else
        acceptance=0;
    end
end

== matlab function ardupilotsailboatold/MATLAB Function6 ==
  data: xw input; yw input; xwp input; y output; ywp input
function y  = distanceToWaypoint(xw,yw,xwp,ywp)
% Calculate distance to waypoint
y = (sqrt((ywp-yw)^2+(xwp-xw)^2))/2;

== matlab function ardupilotsailboatold/MATLAB Function7 ==
  data: wa input; y output; psi input; w output; p output
function [y,w,p]   = apparentWindAngle(wa,psi)
% Calculate Apparent Wind Angle
if psi> pi
    psi= psi-2*pi;
else
    if psi<-pi
    psi=psi+2*pi;
    end
end
awa = psi+ wa;
p=psi;
w= wa;

if abs(awa)<pi/4
    y=1;
else

    y=0;
end

== matlab function ardupilotsailboatold/MATLAB Function8 ==
  data: x1 input; y1 input; u input; y output; us input
function y = controlAngle(x1,y1,u,us)
ys=0;
if x1>=0 && y1>=0
    ys=u;
elseif x1>=0 && y1<=0
        ys=pi-u;
elseif x1==0 && y1>0
        ys=0;
elseif x1==0 && y1<0
        ys=pi;
elseif y1==0 && x1>0
        ys=pi/2;
elseif y1==0 && x1<0
        ys=-pi/2;
elseif x1<0 && y1>0
    ys=-u;
elseif x1<0 && y1<0
    ys=-pi+u;
else
    ys=u;
end
if (ys-us)<-pi
    y = ys+2*pi;
elseif (ys-us)>pi
    y=ys-2*pi;
else
    y=ys;
end

== matlab function ardupilotsailboatold/MATLAB Function9 ==
  data: angle output; dist input; xtrack input; currentState input; tack output; nextState output; windDirection input; wayPointHeading input
function [angle,tack,nextState]  = tackAngle(dist,xtrack,currentState,windDirection,wayPointHeading)
% Calculate when to tack back to waypoint
if dist ~= 0
    angle = atan(xtrack/dist);
else
    angle=0;
end

if windDirection > pi
    windDirection = windDirection - pi;
else
    if windDirection < -pi
        windDirection = windDirection + pi;
    end
end

if wayPointHeading > pi
    wayPointHeading = wayPointHeading - pi;
else
    if wayPointHeading < -pi
        wayPointHeading = wayPointHeading + pi;
    end
end

angle = angle * (180/pi) - (windDirection-wayPointHeading);

% tack == 0 is left tack
% tack == 1 is right tack
switch currentState
    case 0
        tack=0;
        if angle>=45
            nextState=1;
        else
            nextState=0;
        end
    case 1
        tack=1;
        if angle<=-45
            nextState=0;
        else
            nextState=1;
        end

    otherwise
        tack=0;
        nextState=0;

end

== matlab function ardupilotsailboatold/MATLAB Function1 ==
  data: y output; psi input; wind_direction input; alpha_aw output; u input; v input; wind_velocity input; r input; V_aw output
function [y,alpha_aw,V_aw] = sailAngle(psi,wind_direction,u,v,wind_velocity,r)

% CoE of the sail
xs = 0;
ys = 0;
zs = 0.6;
v_t = [ wind_velocity*cos(wind_direction); wind_velocity*sin(wind_direction); 0 ];
R1 = [ cos(-psi) -sin(-psi) 0; sin(-psi) cos(-psi) 0; 0 0 1];
R2 = [ 1 0 0 ; 0 1 0; 0 0 1];
v_tb = R2*R1*v_t; % wind expressed in the body frame
V_in = [ u ; v ; 0 ];
V_awb = v_tb - V_in - cross([0;0;r],[xs;ys;zs]);
V_awu = V_awb(1);
V_awv = V_awb(2);
V_aw = V_awb(1)^2 + V_awb(2)^2;
alpha_aw = atan2(real(V_awv),real(-V_awu));

y=  0.5 * alpha_aw;

== matlab function ardupilotsailboatold/MATLAB Function ==
  data: delta_s input; apparent_velocity input; Xs output; Ys output; Ks output; Ns output; awa output; apparent_wind_angle input; phi input
function [Xs,Ys,Ks,Ns,awa] = sailForce(delta_s,apparent_velocity,apparent_wind_angle,phi)
%Parameters
rho_a = 1.2;
area_sail =0.38;
l1 =0;
l2 = 0;
h1 = 0.6;

% CoE of sail
zs = 0.6;
xs=0;
ys=0;

% Apparent Wind Velocity
awa=apparent_wind_angle;

% Calculate Angle of Attack
alpha = awa-delta_s;


% Calculate Lift and Drag Force
[Cls,Cds] = sailcoef(alpha);
Ls = 0.5*rho_a*area_sail*(apparent_velocity)*Cls;
Ds = 0.5*rho_a*area_sail*(apparent_velocity)*Cds;

% Sail Force components
Xs = (Ls * sin(awa) - Ds * cos(awa));
Ys = (Ls * cos(awa) + Ds * sin(awa));
Ks =- h1 *(Ls * cos(awa) + Ds * sin(awa));
Ns = (-Xs * l2 * sin(delta_s) + Ys*(l1 - l2*cos(delta_s)));

function [Cls,Cds] = sailcoef(attack)
% generate a lookup table for the lift/drag coefficients for the sail
% and compute Cls/Cds from the lookup table using interpolation.

% lookup table
xdata = linspace(-pi,pi,73); % every 5 degrees
xdata = xdata/pi*180;

% lift curve
yldata = [fliplr([0 0.15 0.32 ...
    0.48 0.7 0.94 1.15 1.3 1.28 1.15 1.1 1.05 1 0.9 0.82 0.72 0.68 0.56 0.48 0.32 0.21 0.08 ...
    -0.06 -0.18 -0.3 -0.4 -0.53 -0.64 -0.72 -0.84 -0.95 -1.04 -1.1 -1.14 -1.08 -0.76 0])*(-1) ...
    [0.15 0.32 ...
    0.48 0.7 0.94 1.15 1.3 1.28 1.15 1.1 1.05 1 0.9 0.82 0.72 0.68 0.56 0.48 0.32 0.21 0.08 ...
    -0.06 -0.18 -0.3 -0.4 -0.53 -0.64 -0.72 -0.84 -0.95 -1.04 -1.1 -1.14 -1.08 -0.76 0]];

% drag curve
yddata = [fliplr([0.1 0.12 0.14 ...
    0.16 0.19 0.26 0.35 0.46 0.54 0.62 0.7 0.78 0.9 0.98 1.04 1.08 1.16 1.2 1.24 1.26 ...
    1.28 1.34 1.36 1.37 1.33 1.31 1.28 1.26 1.25 1.2 1.1 1.04 0.88 0.8 0.64 0.38 0.1])...
    [0.12 0.14 ...
    0.16 0.19 0.26 0.35 0.46 0.54 0.62 0.7 0.78 0.9 0.98 1.04 1.08 1.16 1.2 1.24 1.26 ...
    1.28 1.34 1.36 1.37 1.33 1.31 1.28 1.26 1.25 1.2 1.1 1.04 0.88 0.8 0.64 0.38 0.1]];

% fit the input angle of attack into the interval [-pi,pi]
if attack > pi
    attack = mod(attack+pi,2*pi) - pi;
else
    if attack < -pi
        attack = mod(attack-pi,-2*pi) + pi;
    end
end

% interpolation
attack = attack/pi*180;
Cls = interp1(xdata,yldata,attack,'pchip');
Cds = interp1(xdata,yddata,attack,'pchip');

== matlab function ardupilotsailboatold/MATLAB Function2 ==
  data: y output; r input; currentState input; nextState output
function [y,nextState]      = zigzag(r,currentState)
% Beta Reference Angle

switch currentState
    case 0
        if(r==1)
        nextState=1;
        else 
            nextState=0;
        end
        y=-15/180*pi;
    case 1
        if(r==1)
        nextState=0;
        else 
            nextState=1;
        end
        y=15/180*pi;
    otherwise
        y=-15/180*pi;
        nextState=0;
end

== matlab function ardupilotsailboatold/MATLAB Function13 ==
  data: r input; u input; Xr output; v input; Yr output; Kr output; Nr output; delta_r input; delta_r output; alpha_a output
function [Xr,Yr,Kr,Nr,delta_r,alpha_a] = rudderForce(r,u,v,delta_r)
%Parameters
rudder_width = 4;
rudder_length = 20;
rho_w = 1025;
area = rudder_length * rudder_width * 10^(-4);
velocity = sqrt(v^2+u^2);
l4 = 0.48;
h3 = 0.2;
yr = 0;
xr = -0.5;
zr = 0.2;

% Calculate Angle of Attack
v_aru = -u;
v_arv = -v-r;
alpha_ar = atan2(real(v_arv),real(v_aru));
alpha_a = alpha_ar - delta_r;

% Lift and Drag Coeff
[lc, dc] = ruddercoef(alpha_a);


% Calculate Lift and Drag Force
lift_force = 0.5 * rho_w * area * lc * velocity^2 ;
drag_force = 0.5 * rho_w * area * dc * velocity^2 ;

Xr = (lift_force * sin(alpha_ar) - drag_force * cos(alpha_ar));
Yr = (lift_force * cos(alpha_ar) + drag_force * sin(alpha_ar));
Kr =( h3 * ( -lift_force * cos(alpha_ar) - drag_force * sin(alpha_ar)));
Nr = (l4 * (lift_force * cos(alpha_ar) + drag_force * sin(alpha_ar)));


function [Clr,Cdr] = ruddercoef(attack)
% generate a lookup table for the lift/drag coefficients for the sail
% and compute Cls/Cds from the lookup table using interpolation.

% lookup table
xdata = linspace(-pi,pi,73); % every 5 degrees
xdata = xdata/pi*180;

% lift curve
yl = fliplr([0 0.42 0.73 ...
    0.95 1.1 1.165 1.18 1.155 1.12 1.065 1 0.92 0.83 0.72 0.62 0.48 0.33 0.16])*(-1);
yldata = [fliplr([0 0.42 0.73 ...
    0.95 1.1 1.165 1.18 1.155 1.12 1.065 1 0.92 0.83 0.72 0.62 0.48 0.33 0.16 0 yl])*(-1) ...
    [0.42 0.73 ...
    0.95 1.1 1.165 1.18 1.155 1.12 1.065 1 0.92 0.83 0.72 0.62 0.48 0.33 0.16 0 yl]];

% drag curve
yd = fliplr([0 0.03 0.06 ...
    0.1 0.17 0.3 0.48 0.74 0.98 1.18 1.34 1.5 1.65 1.76 1.89 1.97 2.01 2.05]);
yddata = [fliplr([0 0.03 0.06 ...
    0.1 0.17 0.3 0.48 0.74 0.98 1.18 1.34 1.5 1.65 1.76 1.89 1.97 2.01 2.05 2.08 yd])...
    [0.03 0.06 ...
    0.1 0.17 0.3 0.48 0.74 0.98 1.18 1.34 1.5 1.65 1.76 1.89 1.97 2.01 2.05 2.08 yd]];

% fit the input angle of attack into the interval [-pi,pi]
if attack > pi
    attack = mod(attack+pi,2*pi) - pi;
else
    if attack < -pi
        attack = mod(attack-pi,-2*pi) + pi;
    end
end

% interpolation
attack = attack/pi*180;
Clr = interp1(xdata,yldata,attack,'pchip');
Cdr = interp1(xdata,yddata,attack,'pchip');

== matlab function ardupilotsailboatold/MATLAB Function14 ==
  data: beta input; wu output; wv output; wr output; t input
function [wu,wv,wr] = WaveForcesandMoments(beta,t)
% Water density (kg/m^2)
rho = 1025;

% Gravity (m/s^2)
g = 9.81;

% Vessel size (m)
L = 2;
B = 0.125;
T = 0.4;

% Vessels Heading

% Wave Specifications
% amplitude(m)
Ai = 0.4;
% length(m)
lamdai = 5;
% encounter frequency (rads)
omegai = 0.4;
% random phase (rads)
phii = -pi;

% Wave Component
waveC = Ai * (2*pi)/lamdai * sin(omegai*t + phii);

% u Component
wu = (10^(-6)) * rho * g * B * L * T * cos(beta) * waveC;

% v Component
wv = (10^(-6)) * rho * g * B * L * T * sin(beta) * waveC;

% r Component
wr = (10^(-6)) * 1/24 * rho * g * B * L * (L^2 - B^2) * sin(2*beta) * waveC^2;
